simulink library "pmm"  (Simulink 7.0)
undefined symbols (not defined in the file or in its folder): ENUM_PMMMODE_FAULT, ENUM_PMMMODE_IDLE, ENUM_PMMMODE_INITIALIZE, ENUM_PMMMODE_NORMAL, ENUM_PMMMODE_POWER_DOWN, ENUM_PMMMODE_POWER_UP, FALSE, KPMM_ForcePowerDown_flg, KPMM_InitializeWaitTime_s, KPMM_SysPowerModeOvrd_enum, KPMM_SysPowerModeOvrd_flg, slcm, TRUE
settings Model: Creator=jc19  LastModifiedBy=14014

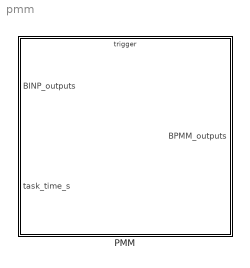
== system pmm ==
  PMM : Subsystem
      settings: RTWSystemCode=Function  RTWFcnNameOpts=Use subsystem name  RTWFileNameOpts=Use subsystem name

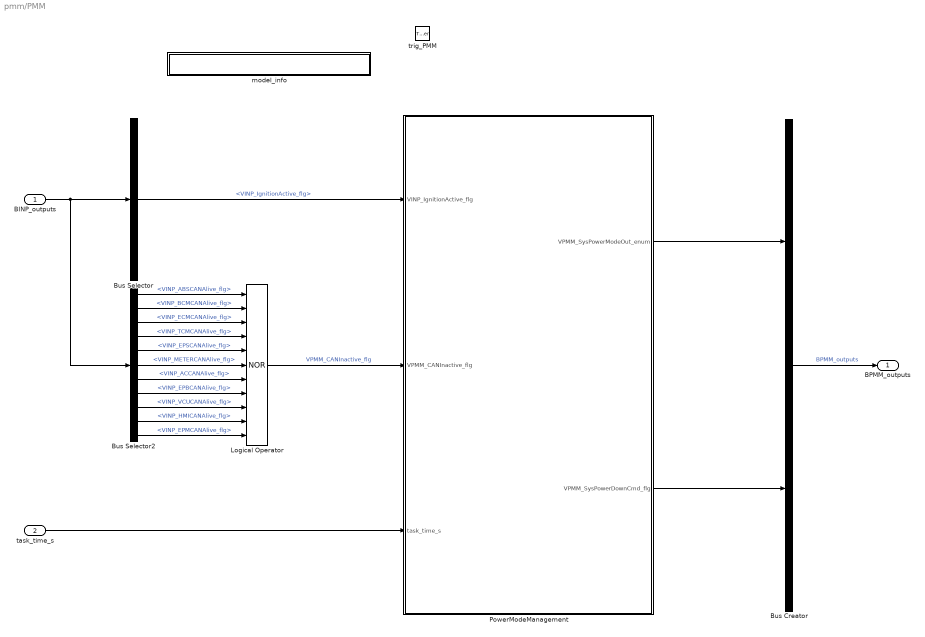
== system pmm/PMM ==
  BINP_outputs : Inport  UseBusObject=on
      settings: BusObject=BINP_outputs
  task_time_s : Inport  Port=2
      settings: BusObject=BINP_outputs
  trig_PMM : TriggerPort  TriggerType=function-call
  Bus Creator : BusCreator  Inputs=2  UseBusObject=on
      settings: BusObject=BPMM_outputs
  Bus Selector : BusSelector  OutputSignals=VINP_IgnitionActive_flg
  Bus Selector2 : BusSelector  OutputSignals=VINP_ABSCANAlive_flg,VINP_BCMCANAlive_flg,VINP_ECMCANAlive_flg,VINP_TCMCANAlive_flg,VINP_EPSCANAlive_flg,VINP_METERCANAlive_flg,VINP_ACCANAlive_flg,VINP_EPBCANAlive_flg,VINP_VCUCANAlive_flg,VINP_HMICANAlive_flg,VINP_EPMCANAlive_flg
  Logical Operator : Logic  Operator=NOR  Inputs=11  AllPortsSameDT=off  OutDataTypeMode=boolean
  PowerModeManagement : Subsystem
  model_info : Subsystem  LoadFcn=slcm LoadBlock;  InitFcn=slcm('UpdateAllCMBlocksInThisModelInit')  mask(CMBlock){InitialSaveTempField=, InitialBlockCM=None, BlockCM=None, Frame=on, SaveTempField=, DisplayStringWithTags=$Id: pmm.mdl 991 2014-11-19 08:50:02Z chimotsai $, MaskDisplayString=$Id: pmm.mdl 991 2014-11-19 08:50:02Z chimotsai $, HorizontalTextAlignment=Center, LeftAlignmentValue=0.5, SourceBlockDiagram=pmm, TagMaxNumber=20, CMTag1=, CMTag2=, CMTag3=, CMTag4=, CMTag5=, CMTag6=, CMTag7=, CMTag8=, CMTag9=, CMTag10=, CMTag11=, CMTag12=, CMTag13=, CMTag14=, CMTag15=, CMTag16=, CMTag17=, CMTag18=, CMTag19=, CMTag20=}
      mask help: This block allows revision control information to be displayed within the model.
      settings: CopyFcn=slcm CopyBlock;  DeleteFcn=slcm Cancel;  PostSaveFcn=slcm('UpdateAllCMBlocksInThisModel')  NameChangeFcn=slcm Rename;  OpenFcn=slcm
      mask Display: text(str2num(LeftAlignmentValue), 0.5, MaskDisplayString, 'HorizontalAlignment', HorizontalTextAlignment)
  BPMM_outputs : Outport  UseBusObject=on
      settings: BusObject=BPMM_outputs
  wires:
  Logical Operator/1 -> PowerModeManagement/2(VPMM_CANInactive_flg)  "VPMM_CANInactive_flg"
  Bus Selector/1 -> PowerModeManagement/1(VINP_IgnitionActive_flg)  "<VINP_IgnitionActive_flg>"
  PowerModeManagement/1(VPMM_SysPowerModeOut_enum) -> Bus Creator/1
  BINP_outputs/1 -> Bus Selector2/1, Bus Selector/1
  Bus Creator/1 -> BPMM_outputs/1  "BPMM_outputs"
  PowerModeManagement/2(VPMM_SysPowerDownCmd_flg) -> Bus Creator/2
  task_time_s/1 -> PowerModeManagement/3(task_time_s)
  Bus Selector2/1 -> Logical Operator/1  "<VINP_ABSCANAlive_flg>"
  Bus Selector2/2 -> Logical Operator/2  "<VINP_BCMCANAlive_flg>"
  Bus Selector2/3 -> Logical Operator/3  "<VINP_ECMCANAlive_flg>"
  Bus Selector2/4 -> Logical Operator/4  "<VINP_TCMCANAlive_flg>"
  Bus Selector2/5 -> Logical Operator/5  "<VINP_EPSCANAlive_flg>"
  Bus Selector2/6 -> Logical Operator/6  "<VINP_METERCANAlive_flg>"
  Bus Selector2/7 -> Logical Operator/7  "<VINP_ACCANAlive_flg>"
  Bus Selector2/8 -> Logical Operator/8  "<VINP_EPBCANAlive_flg>"
  Bus Selector2/9 -> Logical Operator/9  "<VINP_VCUCANAlive_flg>"
  Bus Selector2/10 -> Logical Operator/10  "<VINP_HMICANAlive_flg>"
  Bus Selector2/11 -> Logical Operator/11  "<VINP_EPMCANAlive_flg>"

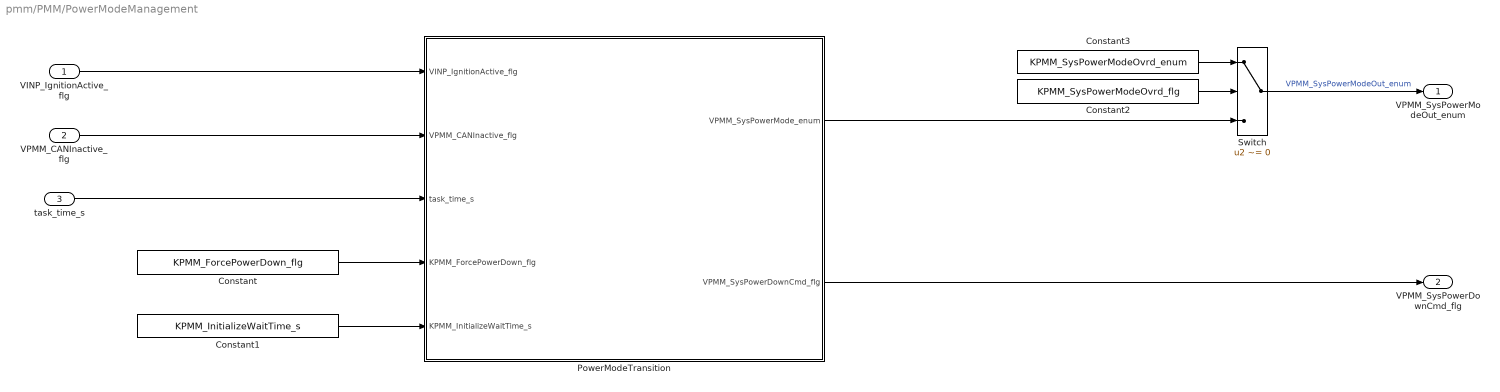
== system pmm/PMM/PowerModeManagement ==
  VINP_IgnitionActive_flg : Inport
  VPMM_CANInactive_flg : Inport  Port=2
  task_time_s : Inport  Port=3
  Constant : Constant  Value=KPMM_ForcePowerDown_flg  OutDataType=sfix(16)  OutScaling=2^0
  Constant1 : Constant  Value=KPMM_InitializeWaitTime_s  OutDataType=sfix(16)  OutScaling=2^0
  Constant2 : Constant  Value=KPMM_SysPowerModeOvrd_flg  OutDataType=sfix(16)  OutScaling=2^0
  Constant3 : Constant  Value=KPMM_SysPowerModeOvrd_enum  OutDataType=sfix(16)  OutScaling=2^0
  PowerModeTransition : Stateflow chart
  Switch : Switch  Criteria=u2 ~= 0  OutDataType=sfix(16)  OutScaling=2^0
  VPMM_SysPowerModeOut_enum : Outport
  VPMM_SysPowerDownCmd_flg : Outport  Port=2
  wires:
  Switch/1 -> VPMM_SysPowerModeOut_enum/1  "VPMM_SysPowerModeOut_enum"
  PowerModeTransition/1(VPMM_SysPowerMode_enum) -> Switch/3
  Constant3/1 -> Switch/1
  Constant2/1 -> Switch/2
  PowerModeTransition/2(VPMM_SysPowerDownCmd_flg) -> VPMM_SysPowerDownCmd_flg/1
  Constant/1 -> PowerModeTransition/4(KPMM_ForcePowerDown_flg)
  VPMM_CANInactive_flg/1 -> PowerModeTransition/2(VPMM_CANInactive_flg)
  VINP_IgnitionActive_flg/1 -> PowerModeTransition/1(VINP_IgnitionActive_flg)
  task_time_s/1 -> PowerModeTransition/3(task_time_s)
  Constant1/1 -> PowerModeTransition/5(KPMM_InitializeWaitTime_s)

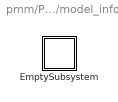
== system pmm/PMM/model_info ==
  EmptySubsystem : Subsystem

== system pmm/PMM/model_info/EmptySubsystem ==

== stateflow chart PMM/PowerModeManagement/PowerModeTransition ==
  state Idle
    entry:
    VPMM_SysPowerMode_enum = ENUM_PMMMODE_IDLE;
    (default) -> (junction 10)
    (junction 10) -> (junction 5) [order 2]
    (junction 6) -> (junction 5)
    Idle -> (junction 10) [order 1]
    (junction 10) -> (junction 7) [order 1] : [VPMM_CANInactive_flg]
    (junction 7) -> (junction 6) : {VPMM_SysPowerDownCmd_flg = TRUE;}
  state Normal
    entry:
    VPMM_SysPowerMode_enum = ENUM_PMMMODE_NORMAL;
    Normal -> (junction 8) [order 1]
    (default) -> (junction 8) : {VPMM_InitializeTime_s = 0;
        | VPMM_SysPowerDownCmd_flg = FALSE;}
    (junction 8) -> (junction 9) : {VPMM_InitializeTime_s = VPMM_InitializeTime_s+task_time_s;}
  Normal -> Idle [order 1] : [((VPMM_InitializeTime_s > KPMM_InitializeWaitTime_s) && ...
      | ((!VINP_IgnitionActive_flg) && VPMM_CANInactive_flg)) ||...
      | KPMM_ForcePowerDown_flg]
  (default) -> Normal
  Idle -> Normal [order 1] : [VINP_IgnitionActive_flg]
  data: VINP_IgnitionActive_flg input inherited; VPMM_SysPowerMode_enum output uint8; TRUE parameter inherited; FALSE parameter inherited; VPMM_SysPowerDownCmd_flg output boolean; ENUM_PMMMODE_INITIALIZE parameter inherited; ENUM_PMMMODE_POWER_UP parameter inherited; ENUM_PMMMODE_NORMAL parameter inherited; ENUM_PMMMODE_POWER_DOWN parameter inherited; ENUM_PMMMODE_IDLE parameter inherited; ENUM_PMMMODE_FAULT parameter inherited; VPMM_CANInactive_flg input inherited; task_time_s input inherited; KPMM_ForcePowerDown_flg input inherited; KPMM_InitializeWaitTime_s input inherited; VPMM_InitializeTime_s local double
